simulink model "threephase_rlc_motor"  (R2014a)
settings: Solver=ode23tb  StartTime=0.0  StopTime=10  MaxStep=1e-3  RelTol=1e-4
undefined symbols (not defined in the file or in its folder): D1, Delta
libraries: powerlib x11
settings Model: Creator=cosorio  LastModifiedBy=cosorio

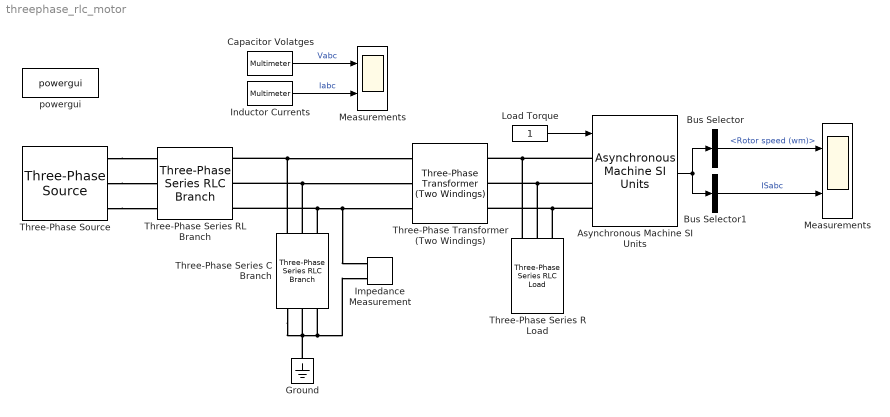
== system threephase_rlc_motor ==
  Asynchronous Machine SI Units : powerlib/Machines/Asynchronous Machine SI Units  PresetModel=No  MechanicalLoad=Torque Tm  ShowDetailedParameters=on  RotorType=Squirrel-cage  ReferenceFrame=Rotor  Units=SI  MeasurementBus=off  NominalParameters=[3.73e+04 460 60]  Stator=[0.09961 0.000867]  Rotor=[0.05837 0.000867]  Cage1=[ 0.022 0.226/377]  Cage2=[ 0.022 0.226/377]  Lm=0.03039  Mechanical=[0.4 0.02187 2]  PolePairs=2  InitialConditions=[1 0 0 0 0 0 0 0]  SimulateSaturation=off  Saturation=[14.03593122, 27.81365428, 53.79336849, 72.68890987, 97.98006896, 148.6815601, 215.7428561, 302.9841135, 420.4778367 ; 230, 322, 414, 460, 506, 552, 598, 644, 690]  LoadFlowParameters=1492000  TsPowergui=0  TsBlock=-1  IterativeModel=Trapezoidal non iterative  Pmec=0
  Bus Selector : BusSelector  OutputSignals=Mechanical.Rotor speed (wm)
  Bus Selector1 : BusSelector  OutputSignals=Stator measurements.Stator current is_a (A),Stator measurements.Stator current is_b (A),Stator measurements.Stator current is_c (A)  OutputAsBus=on
  Capacitor Volatges : powerlib/Measurements/Multimeter  PhasorSimulation=off  OutputType=Complex  sel=[1 2 3]  L=6  Gain=[1 1 1]  yselected={'Ub1: Three-Phase Series C Branch','Ub2: Three-Phase Series C Branch','Ub3: Three-Phase Series C Branch'};  PSBOutputType=1  PSBequivalent=0  AxesSetting=[0,0.1,-100,100]  Display=0  SavedBlockNames=-11
  Ground : powerlib/Elements/Ground  LConnTagsString=a
  Impedance Measurement : powerlib/Measurements/Impedance Measurement  LConnTagsString=+|-  Factor=1
  Inductor Currents : powerlib/Measurements/Multimeter  PhasorSimulation=off  OutputType=Complex  sel=[4 5 6]  L=6  Gain=[1 1 1]  yselected={'Ib1: Three-Phase Series RL Branch','Ib2: Three-Phase Series RL Branch','Ib3: Three-Phase Series RL Branch'};  PSBOutputType=1  PSBequivalent=0  AxesSetting=[0,0.1,-100,100]  Display=0  SavedBlockNames=-11
  Load Torque : Constant
  Measurements : Scope  NumInputPorts=2
      settings: YMin=-40000~-100  YMax=40000~100
  "Measurements " : Scope  NumInputPorts=2
      settings: YMin=0~-200  YMax=200~200
  Three-Phase Series C Branch : powerlib/Elements/Three-Phase Series RLC Branch  LConnTagsString=A|B|C  RConnTagsString=A|B|C  BranchType=C  Resistance=1  Inductance=1e-3  Capacitance=1e-6  Measurements=Branch voltages
  Three-Phase Series R Load : powerlib/Elements/Three-Phase Series RLC Load  LConnTagsString=A|B|C  Configuration=Y (grounded)  NominalVoltage=1000  NominalFrequency=60  ActivePower=10e3  InductivePower=0  CapacitivePower=0  Measurements=None  LoadType=constant Z
  Three-Phase Series RL Branch : powerlib/Elements/Three-Phase Series RLC Branch  LConnTagsString=A|B|C  RConnTagsString=A|B|C  BranchType=RL  Resistance=1  Inductance=1e-3  Capacitance=1e-6  Measurements=Branch currents
  Three-Phase Transformer (Two Windings) : powerlib/Elements/Three-Phase Transformer (Two Windings)  Winding1Connection=Yg  UNITS=pu  NominalPower=[ 250e6 , 60 ]  Winding1=[ 735e3 , 0.002 , 0.08 ]  Winding2Connection=Delta (D1)  Winding2=[ 315e3 , 0.002 , 0.08 ]  SetSaturation=off  Rm=500  Lm=500  Saturation=[ 0,0 ; 0.0024,1.2 ; 1.0,1.52 ]  Hysteresis=off  DataFile='hysteresis'  SetInitialFlux=off  InitialFluxes=[ 0.8 , -0.8 , 0.7 ]  Measurements=None  MoreParameters=off  BreakLoop=off  DataType=off  TransfoNumber=1
  Three-Phase Source : powerlib/Electrical Sources/Three-Phase Source  Voltage=25e3  PhaseAngle=0  Frequency=60  InternalConnection=Yg  SpecifyImpedance=on  Resistance=0.8929  Inductance=16.58e-3  ShortCircuitLevel=100e6  BaseVoltage=25e3  XRratio=7  BusType=swing  Pref=0  Qref=0  Qmin=-inf  Qmax=inf
  powergui : powerlib/powergui  Priority=1  SimulationMode=Continuous  SolverType=Tustin  SampleTime=50e-6  frequency=60  SPID=off  DisableSnubberDevices=off  DisableRonSwitches=off  DisableVfSwitches=off  SwTol=0  Interpol=off  DisplayEquations=off  Ts=0  methode=off  frequencyindice=60  Pbase=100e6  ErrMax=1e-4  Iterations=50  UnitsV=kV  UnitsW=MW  FunctionMessages=off  echomessages=off  HookPort=off  EnableUseOfTLC=off  x0status=blocks  RestoreLinks=warning  ResistiveCurrentMeasurement=off  Frange=logspace(0,4,100)  Ylog=on  Xlog=on  ShowGrid=off  save=off  variable=ZData  structure=0  ZoomFFT=off  StartTime=0.0  cycles=1  DisplayStyle=1  fundamental=60  FreqAxis=off  MaxFrequency=1000  frequencyindicesteady=1  RmsSteady=1  display=off
  wires:
  Inductor Currents/1 -> Measurements/2  "Iabc"
  Capacitor Volatges/1 -> Measurements/1  "Vabc"
  Load Torque/1 -> Asynchronous Machine SI Units/1
  Asynchronous Machine SI Units/1 -> Bus Selector1/1, Bus Selector/1
  Bus Selector1/1 -> "Measurements "/2  "ISabc"
  Bus Selector/1 -> "Measurements "/1  "<Rotor speed (wm)>"
  connections:
  Three-Phase Source/RConn1 -- Three-Phase Series RL Branch/LConn1
  Three-Phase Source/RConn2 -- Three-Phase Series RL Branch/LConn2
  Three-Phase Source/RConn3 -- Three-Phase Series RL Branch/LConn3
  Three-Phase Series C Branch/LConn1 -- Three-Phase Series RL Branch/RConn1 -- Three-Phase Transformer (Two Windings)/LConn1
  Three-Phase Series C Branch/LConn2 -- Three-Phase Series RL Branch/RConn2 -- Three-Phase Transformer (Two Windings)/LConn2
  Three-Phase Series C Branch/LConn3 -- Impedance Measurement/LConn1 -- Three-Phase Transformer (Two Windings)/LConn3 -- Three-Phase Series RL Branch/RConn3
  Ground/LConn1 -- Impedance Measurement/LConn2 -- Three-Phase Series C Branch/RConn3 -- Three-Phase Series C Branch/RConn1 -- Three-Phase Series C Branch/RConn2
  Asynchronous Machine SI Units/LConn1 -- Three-Phase Transformer (Two Windings)/RConn1 -- Three-Phase Series R Load/LConn1
  Asynchronous Machine SI Units/LConn3 -- Three-Phase Series R Load/LConn3 -- Three-Phase Transformer (Two Windings)/RConn3
  Asynchronous Machine SI Units/LConn2 -- Three-Phase Series R Load/LConn2 -- Three-Phase Transformer (Two Windings)/RConn2
